simulink model "model_mussels"  (R2014b)
settings: Solver=ode45  SolverMode=SingleTasking  StartTime=0.0  StopTime=30  RelTol=1e-3
values from neighbouring files (symbols this model uses):
  adapt = 1    [init.m]    (also in init_model.m; init_mussels.m; init_mussels_2.m; init_mussels_konfiguracija_blizu.m)
  K = 0.02    [init.m]    (also in init_model.m; init_mussels.m; init_mussels_2.m; init_mussels_konfiguracija_blizu.m)
  pos_0 = zeros(3,n)    [init_mussels.m]    (also in init_mussels_2.m; init_mussels_konfiguracija_blizu.m = [1, 3, 3, 1, 2; init_mussels_konfiguracija_daleko.m = [10, 20, 20, 10, 15; init_mussels_konfiguracija_srednje.m = [0 0 0 0 1)
  sigma_0 = [ 0    0.7   0    0    0 ... (first row only)    [init.m]    (also in init_model.m = zeros(M,M); init_mussels.m = zeros(n,n); init_mussels_2.m; init_mussels_konfiguracija_blizu.m = [ 0    0.7   0.4    0.6    0.5)
  zeta_0 = zeros(n,n)    [init.m]    (also in init_model.m = zeros(M,M); init_mussels.m; init_mussels_2.m; init_mussels_konfiguracija_blizu.m)
settings Model: CovSFcnEnable=on  Creator=Marta_2805  LastModifiedBy=Annie
settings OptimizationCC: BlockReduction=off  BooleanDataType=off  UseDivisionForNetSlopeComputation=off  SimCompilerOptimization=off
settings DebuggingCC: SaveWithParameterizedLinksMsg=none  UnderspecifiedInitializationDetection=Classic  MergeDetectMultiDrivingBlocksExec=none  SignalResolutionControl=TryResolveAllWithWarning  SolverPrmCheckMsg=none  FrameProcessingCompatibilityMsg=error
settings HardwareCC: TargetUnknown=on
settings RTWCC: RTWCompilerOptimization=off

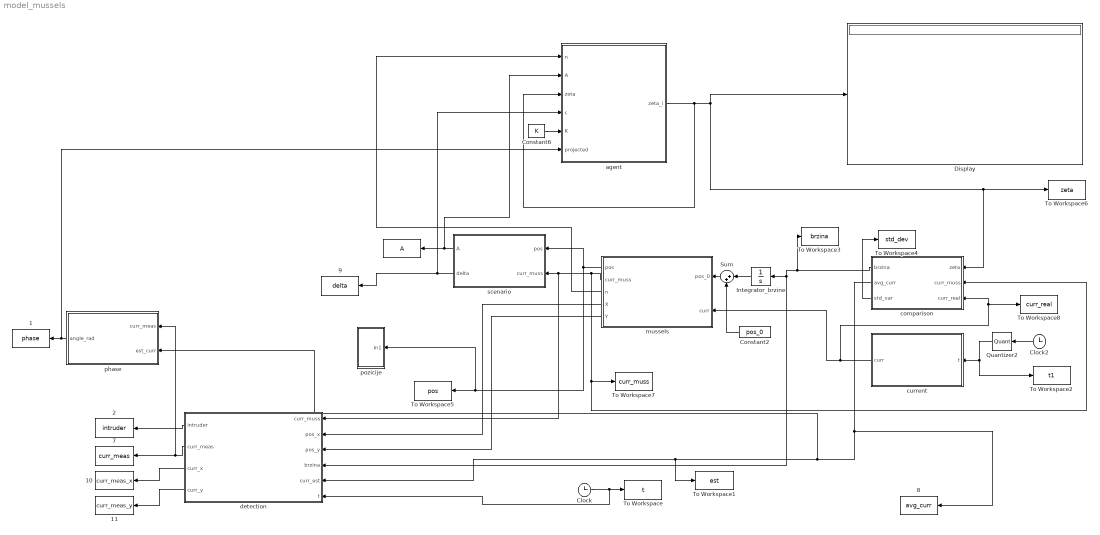
== system model_mussels ==
  " 1" : ToWorkspace  VariableName=phase  SampleTime=-1
  " 10" : ToWorkspace  VariableName=curr_meas_x  SampleTime=-1
  " 11" : ToWorkspace  VariableName=curr_meas_y  SampleTime=-1
  " 2" : ToWorkspace  VariableName=intruder  SampleTime=-1
  " 7" : ToWorkspace  VariableName=curr_meas  SampleTime=-1
  " 8" : ToWorkspace  VariableName=avg_curr  SampleTime=-1
  " 9" : ToWorkspace  VariableName=delta  SampleTime=-1
  " " : ToWorkspace  VariableName=A  SampleTime=-1
  Clock : Clock
  Clock2 : Clock
      settings: Decimation=1000
  Constant2 : Constant  Value=pos_0
  Constant6 : Constant  Value=K
  Display : Display
  Integrator_brzine : Integrator  InitialCondition=[1 1 1 1 1;1 1 1 1 1;1 1 1 1 1]
  Quantizer2 : Quantizer  QuantizationInterval=1
  Sum : Sum  Inputs=|++
  To Workspace : ToWorkspace  VariableName=t  SampleTime=-1
  To Workspace1 : ToWorkspace  VariableName=est  SampleTime=-1
  To Workspace2 : ToWorkspace  VariableName=t1  SampleTime=-1
  To Workspace3 : ToWorkspace  VariableName=brzina  SampleTime=-1
  To Workspace4 : ToWorkspace  VariableName=std_dev  SampleTime=-1
  To Workspace5 : ToWorkspace  VariableName=pos  SampleTime=-1
  To Workspace6 : ToWorkspace  VariableName=zeta  SampleTime=-1
  To Workspace7 : ToWorkspace  VariableName=curr_muss  SampleTime=-1
  To Workspace8 : ToWorkspace  VariableName=curr_real  SampleTime=-1
  "agent " : Subsystem
  comparison : MATLAB Function  TreatAsAtomicUnit=on
  current : MATLAB Function  TreatAsAtomicUnit=on
  detection : MATLAB Function  TreatAsAtomicUnit=on
  mussels : MATLAB Function  TreatAsAtomicUnit=on
  phase : MATLAB Function  TreatAsAtomicUnit=on
  pozicije : Subsystem
  scenario : MATLAB Function  TreatAsAtomicUnit=on
  wires:
  Constant6/1 -> "agent "/5(K)
  "agent "/1(zeta_i) -> Display/1, comparison/1(zeta), To Workspace6/1, "agent "/3(zeta)
  mussels/1(pos) -> scenario/1(pos), pozicije/1(In1), To Workspace5/1
  scenario/1(A) -> " "/1, "agent "/2(A)
  mussels/3(n) -> "agent "/1(n)
  Sum/1 -> mussels/1(pos_0)
  Clock/1 -> detection/6(t), To Workspace/1
  comparison/1(brzina) -> To Workspace3/1, detection/4(brzina), Integrator_brzine/1
  Constant2/1 -> Sum/2
  Integrator_brzine/1 -> Sum/1
  mussels/2(curr_muss) -> To Workspace7/1, comparison/2(curr_muss), detection/1(curr_muss), scenario/2(curr_muss)
  Clock2/1 -> Quantizer2/1
  Quantizer2/1 -> To Workspace2/1, current/1(t)
  current/1(curr) -> To Workspace8/1, comparison/3(curr_real), mussels/2(curr)
  scenario/2(delta) -> " 9"/1, "agent "/4(c)
  mussels/5(Y) -> detection/3(pos_y)
  comparison/2(avg_curr) -> phase/2(est_curr), To Workspace1/1, detection/5(curr_est), " 8"/1
  detection/1(intruder) -> " 2"/1
  detection/2(curr_meas) -> " 7"/1, phase/1(curr_meas)
  phase/1(angle_rad) -> "agent "/6("projected "), " 1"/1
  mussels/4(X) -> detection/2(pos_x)
  comparison/3(std_var) -> To Workspace4/1
  detection/3(curr_x) -> " 10"/1
  detection/4(curr_y) -> " 11"/1

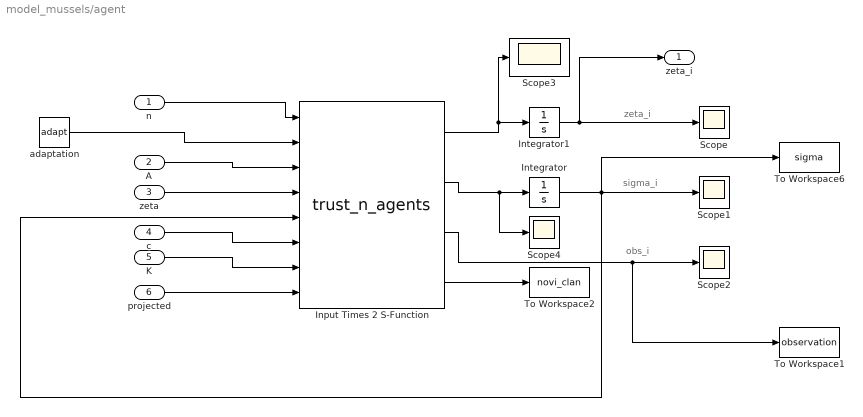
== system model_mussels/agent  ==
  note: obs_i
  note: sigma_i
  note: zeta_i
  n : Inport
  A : Inport  Port=2
  zeta : Inport  Port=3
  c : Inport  Port=4
  K : Inport  Port=5
  "projected " : Inport  Port=6
  Input Times 2 S-Function : S-Function  FunctionName=trust_n_agents  EnableBusSupport=off
  Integrator : Integrator  InitialCondition=sigma_0
  Integrator1 : Integrator  InitialCondition=zeta_0
  Scope{,1..4} (5 alike) : Scope
      Scope settings: TimeRange=20  YMin=0.25  YMax=0.95
      Scope2 settings: YMin=0  YMax=0.2  SaveName=ScopeData2
      Scope3 settings: TimeRange=20  YMin=0.25  YMax=0.95  SaveName=ScopeData3
      Scope4 settings: TimeRange=20  YMin=0.25  YMax=0.95  SaveName=ScopeData4
  To Workspace1 : ToWorkspace  VariableName=observation  SampleTime=-1
  To Workspace2 : ToWorkspace  VariableName=novi_clan  SampleTime=-1
  To Workspace6 : ToWorkspace  VariableName=sigma  SampleTime=-1
  adaptation : Constant  Value=adapt
  zeta_i : Outport
  wires:
  Integrator/1 -> Input Times 2 S-Function/5, To Workspace6/1, Scope1/1
  c/1 -> Input Times 2 S-Function/6
  K/1 -> Input Times 2 S-Function/7
  Input Times 2 S-Function/2 -> Scope4/1, Integrator/1
  Input Times 2 S-Function/1 -> Scope3/1, Integrator1/1
  Input Times 2 S-Function/3 -> To Workspace1/1, Scope2/1
  n/1 -> Input Times 2 S-Function/1
  adaptation/1 -> Input Times 2 S-Function/2
  zeta/1 -> Input Times 2 S-Function/4
  A/1 -> Input Times 2 S-Function/3
  Integrator1/1 -> zeta_i/1, Scope/1
  "projected "/1 -> Input Times 2 S-Function/8
  Input Times 2 S-Function/4 -> To Workspace2/1

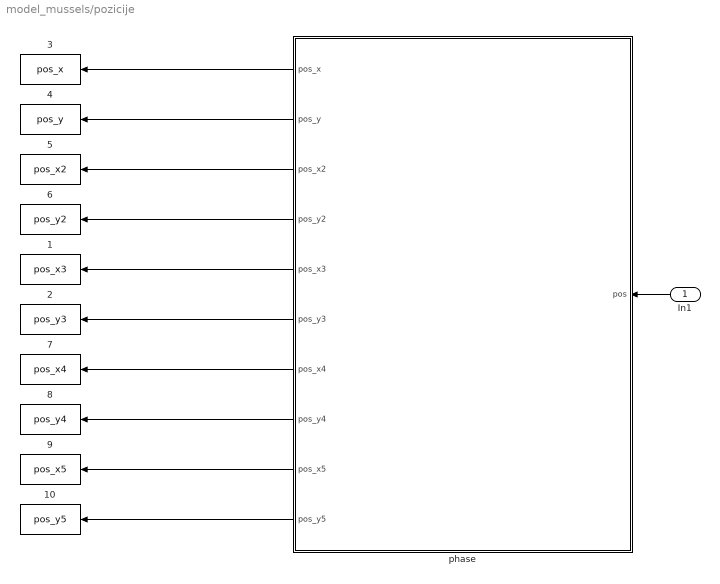
== system model_mussels/pozicije ==
  In1 : Inport
  " 1" : ToWorkspace  VariableName=pos_x3  SampleTime=-1
  " 10" : ToWorkspace  VariableName=pos_y5  SampleTime=-1
  " 2" : ToWorkspace  VariableName=pos_y3  SampleTime=-1
  " 3" : ToWorkspace  VariableName=pos_x  SampleTime=-1
  " 4" : ToWorkspace  VariableName=pos_y  SampleTime=-1
  " 5" : ToWorkspace  VariableName=pos_x2  SampleTime=-1
  " 6" : ToWorkspace  VariableName=pos_y2  SampleTime=-1
  " 7" : ToWorkspace  VariableName=pos_x4  SampleTime=-1
  " 8" : ToWorkspace  VariableName=pos_y4  SampleTime=-1
  " 9" : ToWorkspace  VariableName=pos_x5  SampleTime=-1
  phase : MATLAB Function  TreatAsAtomicUnit=on
  wires:
  phase/3(pos_x2) -> " 5"/1
  phase/4(pos_y2) -> " 6"/1
  phase/2(pos_y) -> " 4"/1
  phase/1(pos_x) -> " 3"/1
  In1/1 -> phase/1(pos)
  phase/5(pos_x3) -> " 1"/1
  phase/6(pos_y3) -> " 2"/1
  phase/7(pos_x4) -> " 7"/1
  phase/8(pos_y4) -> " 8"/1
  phase/9(pos_x5) -> " 9"/1
  phase/10(pos_y5) -> " 10"/1

== matlab function model_mussels/scenario ==
  data: pos input; curr_muss input; A output; delta output
function [A, delta]  = scenario(pos, curr_muss)
%#codegen
%radijus komunikacije
r = 5;

%racunanje delte
delta=zeros(5);
error=0;

n=length(pos);
%[m,n] = size(pos);
%inicijalizacija matrice A
A=zeros(n);

for i = 1:n
    for j = 1:n
        %odredivanje udaljenosti izmedju musula - prvo x, y, pa z
        distance = sqrt((pos(1,i)-pos(1,j))^2 + (pos(2,i)-pos(2,j))^2+(pos(3,i)-pos(3,j))^2);
        
        %provjera mogu li komunicirati
        if distance < r
            
            %element ne komunicira sam sa sobom
            if i == j
                A(i,j) = 0;
            else
                A(i,j) = 1;
            end
                        
        else
            A(i,j) = 0;
        end
        
    end
       
end

for i =1:5
    for j=1:5
        
        error = abs(sqrt(curr_muss(i,1)^2+curr_muss(i,2)^2)-sqrt(curr_muss(j,1)^2+curr_muss(j,2)^2));
        delta(i,j)=error;
        
    end
end

delta = delta.*A;

end

== matlab function model_mussels/mussels ==
  data: pos_0 input; pos output; curr_muss output; curr input; n output; X output; Y output
function [pos, curr_muss, n, X, Y] = mussels (pos_0, curr)
%#codegen
%u inpute bi trebalo dodati koordinate, deltu i zetu?

n=5;
pos = pos_0;

%varijable za struju
curr_ag=0;
curr_muss = zeros(n,2);
k = zeros (n,2);

X = pos(1,1);
Y = pos(2,1);
Z = pos(3,1);

%mjerenja

%agent 5 mjeri pogresnu struju
if n==5

%0.0309 0.4755; 0.0309, 0.4755; 0.0309, 0.4755
    k = [1 1; 1 1; 0.0309 0.4755; 0.0309, 0.4755; 0.0309, 0.4755];
    curr_ag = [curr; curr; curr; curr; curr];

end

curr_muss = k.*curr_ag;

end

== matlab function model_mussels/current ==
  data: curr output; t input
function curr = current (t)
%#codegen

alfa_rad =0;
v_x=0;
v_y=0;
v = 0;

%% kod za promjenjivu struju
%{
persistent brojac;
if isempty(brojac)
    brojac = 0;
end

persistent alfa;
if isempty(alfa)
    alfa = 0;
end


if t<20
    
    if mod(t, 3) == 0 & floor(t/3) > brojac
        
        brojac = brojac +1;
        alfa = alfa+3;
        
        if mod(alfa, 360) == 0
            alfa=0;
        end    
    end
end


alfa_rad = alfa * pi / 180;
v=1;
v_x= v * sin(alfa_rad);
v_y= v * cos(alfa_rad);
%}

curr=[1 1];
        
end

== matlab function model_mussels/comparison ==
  data: zeta input; brzina output; curr_muss input; avg_curr output; curr_real input; std_var output
function [brzina, avg_curr, std_var] = comparison (zeta,curr_muss, curr_real)
%#codegen

%prosjecna izracunata struja iz povjerenja i struja musula
avg_curr=[0 0]; 

std_var=std(zeta);

brzina=zeros(3,5);
threshold = 1e-1; 
threshold_zeta=[0.01, 0.01, 0.01, 0.01, 0.01];
threshold_zeta_change=[0.05, 0.05, 0.05, 0.05, 0.05];

a=zeros(1,5);
b=zeros(1,5);
suma_x=0;
suma_y=0;

%komponente za leadera
average_x=0;
average_y=0;

%prava struja
k = [1 1; 1 1; 1 1; 1 1; 1 1];
curr_r = [curr_real; curr_real; curr_real; curr_real; curr_real];

curr_re = k.*curr_r;

maxNum = 100;
persistent num;
if isempty(num)
    num = 1;
end

persistent queue;
if isempty(queue)
    queue = zeros(maxNum, 5);
end


queue(mod(num, maxNum) + 1, :) = zeta(1,:);
num = num + 1;
std_zeta_100 = std(queue);


%% racunanje estimirane struje ukljucujuci sve agente
%{
%racunanje prosjecnih struja svakog agenta za x komponentu struje
for i=1:5
    
    a(i) = average_curr(i,1,zeta,curr_muss);
    
end

suma_x=sum(a);
average_x=suma_x/5;

%racunanje prosjecnih struja svakog agenta za y komponentu struje
for i=1:5
    
    b(i) = average_curr(i,2,zeta,curr_muss);
    
end


suma_y=sum(b);
average_y=suma_y/5;

avg_curr = [average_x average_y];
%}
%% racunanje estimirane struje promatrajuci samo leadera

%trazenje leadera (leader je I)

if (all(abs(std_var) <= threshold_zeta) & all(std_zeta_100 <= threshold_zeta_change))
    
    [M,I] = max(max(zeta));
    avg_curr = [curr_muss(I,1) curr_muss(I,2)];
    
end

%{
for i=1:5
    
    avg_leader_x(i) = average_curr_leader(zeta, curr_muss, I, 1);
  
end

suma_x=sum(avg_leader_x);
average_x=suma_x/5;

%racunanje prosjecnih struja svakog agenta za y komponentu struje
for i=1:5
    
    avg_leader_y(i) = average_curr_leader(zeta, curr_muss, I, 2);
    
end

suma_y=sum(avg_leader_y);
average_y=suma_y/5;

%}

%% postavljanje brzine

%zeljeni smjer struje
wanted =[0.0309, 0.4755];
%wanted =[0.7, 0.2];


%ako je zeljena jednaka estimiranoj struji, mussule se pocinju kretati
if (all(abs(wanted - avg_curr)<= threshold) & all(abs(std_var) <= threshold_zeta) & all(std_zeta_100 <= threshold_zeta_change))
    
       brzina = [curr_re(1) curr_re(1) curr_re(1) curr_re(1) curr_re(1);
                 curr_re(2) curr_re(2) curr_re(2) curr_re(2) curr_re(2);
                 0 0 0 0 0];
else
    brzina = zeros(3,5);
end

v_x=brzina(1,1);
v_y=brzina(2,1);

end

%funkcija koja racuna prosjecnu struju agenta, u smjeru komponente_struje,
%uz predanu matricu povjerenja zeta te struje_musula (to je struja koju
%musule mjere s nekom greskom ili ne)
function c = average_curr(agent, komponenta_struje, zeta, struja_musula)

zbroj_zeta =0;
umnozak =0;
c=0;

for i =1:5
           
    umnozak = umnozak+(zeta(i, agent)*struja_musula(i,komponenta_struje));
    zbroj_zeta=zbroj_zeta+zeta(i, agent);
        
end

c=umnozak/zbroj_zeta;

end

== matlab function model_mussels/detection ==
  data: curr_muss input; pos_x input; pos_y input; brzina input; intruder output; curr_est input; t input; curr_meas output; curr_x output; curr_y output
function [intruder, curr_meas, curr_x, curr_y]    = detection (curr_muss, pos_x,pos_y, brzina, curr_est, t)

threshold = 1e-1;


provjera_jednakosti=2;

intruder =0;

razlika = zeros(3,5);

persistent curr;
if isempty(curr)
    curr = [0 0];
end

persistent brojac;
if isempty(brojac)
    brojac = 0;
end

persistent index;
if isempty(index)
    index = 0;
end

persistent x1;
if isempty(x1)
    x1 = 0;
end

persistent x2;
if isempty(x2)
    x2 = 0;
end

persistent y1;
if isempty(y1)
    y1 = 0;
end

persistent y2;
if isempty(y2)
    y2 = 0;
end

persistent t1;
if isempty(t1)
    t1 = 0;
end

persistent t2;
if isempty(t2)
    t2 = 0;
end

brojac = brojac + 1;
if (mod(brojac,500) == 0)
    %provjera je li brzina veca od 0
    m=zeros(3,5);

    if all(abs(brzina(1,:))) > threshold && all(abs(brzina(2,:))) > threshold
        c = 0;
        
    else
        curr = [0 0];
        c = 1;
    end
    
    

        %izdvajanje pozicija musule 1

        x1 = x2;
        y1 = y2;
        t1 = t2;

        x2 = pos_x(1);
        y2 = pos_y(1);
        t2 = t;

        %racunanje izmjerene brzine u x i y smjeru
        if (x1 & x2 & y1 &y2 & t1 &t2)
            curr_meas_x = sqrt((x2-x1)^2)/(t2-t1);
            curr_meas_y = sqrt((y2-y1)^2)/(t2-t1);
            curr = [curr_meas_x, curr_meas_y];
        end
    
        %provjera micu li se u zeljenom smjeru
        if all(abs(curr - curr_est)<= threshold)
            provjera_jednakosti=1;

        else
            provjera_jednakosti=0;
        end

        %ovaj dio treba provjeravati koji agent grijesi ako se micu u krivom
        %smjeru - grijesi agent s najmanjim povjerenjem
        if provjera_jednakosti == 0
            intruder = 1;
        end
end

curr_meas = [curr(1) curr(2)];

curr_x=curr(1);
curr_y=curr(2);


end

== matlab function model_mussels/phase ==
  data: angle_rad output; curr_meas input; est_curr input
function angle_rad  = phase (curr_meas, est_curr)
%#codegen



if (curr_meas(1) == 0 & curr_meas(2) == 0) || (est_curr(1) == 0 & est_curr(2) == 0)
    angle = 0;
    angle_rad=0;

else
    angle_rad = anglevec(curr_meas, est_curr);
    angle = angle_rad*180/pi;
end
    
end

function [alfarad] = anglevec(u, v)

threshold = 1e-1;

    if all(abs(u - v)<= threshold)
     
        alfarad=0;
        
    else
        
        CosTheta = dot(u,v)/(norm(u)*norm(v));
        alfarad = acos(CosTheta);

    end

end

== matlab function model_mussels/pozicije/phase ==
  data: pos_x output; pos input; pos_y output; pos_x2 output; pos_y2 output; pos_x3 output; pos_y3 output; pos_x4 output; pos_y4 output; pos_x5 output; pos_y5 output
function [pos_x, pos_y, pos_x2, pos_y2, pos_x3, pos_y3, pos_x4, pos_y4, pos_x5, pos_y5]  = positions (pos)
%#codegen

pos_x = pos(1,1);

pos_y = pos(2,1);

pos_x2 = pos(1,2);

pos_y2 = pos(2,2);

pos_x3 = pos(1,3);

pos_y3 = pos(2,3);

pos_x4 = pos(1,4);

pos_y4 = pos(2,4);

pos_x5 = pos(1,5);

pos_y5 = pos(2,5);

end
